simulink model "Valve"  (R2024a)
settings: Solver=ode1be  StartTime=0.0  StopTime=10.0  FixedStep=0.001  RelTol=1e-3
settings Model: Creator=ojklem  LastModifiedBy=ojklem

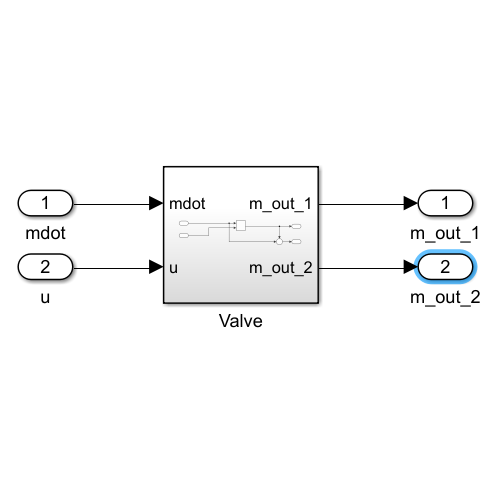
[thumbnail: Simulink's stored preview of the top-level diagram]
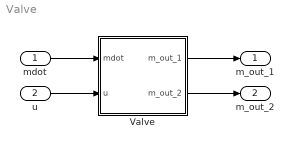
== system Valve ==
  mdot : Inport
  u : Inport  Port=2
  Valve : Subsystem
  m_out_1 : Outport
  m_out_2 : Outport  Port=2
  wires:
  mdot/1 -> Valve/1(mdot)
  u/1 -> Valve/2(u)
  Valve/1(m_out_1) -> m_out_1/1
  Valve/2(m_out_2) -> m_out_2/1

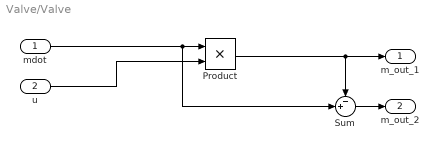
== system Valve/Valve ==
  mdot : Inport
  u : Inport  Port=2
  Product : Product
  Sum : Sum  Inputs=-+|
  m_out_1 : Outport
  m_out_2 : Outport  Port=2
  wires:
  mdot/1 -> Sum/2, Product/1
  Product/1 -> Sum/1, m_out_1/1
  u/1 -> Product/2
  Sum/1 -> m_out_2/1
